simulink model "polygone_task"  (R2016a)
settings: Solver=FixedStepAuto  StartTime=0.0  StopTime=inf  FixedStep=1  RelTol=1e-3
undefined symbols (not defined in the file): Header
libraries: robotlib x3
settings Model: Creator=root  LastModifiedBy=root
settings OptimizationCC: OptimizeModelRefInitCode=on  LifeSpan=Inf  MaxStackSize=64
settings HardwareCC: ProdBitPerPointer=32  ProdLargestAtomicFloat=None  ProdIntDivRoundTo=Undefined  ProdEndianess=Unspecified  ProdWordSize=32  ProdHWDeviceType=Generic->Unspecified (assume 32-bit Generic)
settings RTWCC: SystemTargetFile=ert.tlc  HardwareBoard=Robot Operating System (ROS)  TemplateMakefile=ert_default_tmf  GenerateReport=on  Toolchain=Catkin  IncludeHyperlinkInReport=on  LaunchReport=on  TargetLang=C++  GenerateTraceInfo=on  GenerateTraceReport=on  GenerateTraceReportSl=on  GenerateTraceReportSf=on  GenerateTraceReportEml=on
settings CodeAppCC: ForceParamTrailComments=on  IgnoreCustomStorageClasses=off  OperatorAnnotations=on  SimulinkDataObjDesc=on  SFDataObjDesc=on  MATLABFcnDesc=on  InsertBlockDesc=on  MATLABSourceComments=on

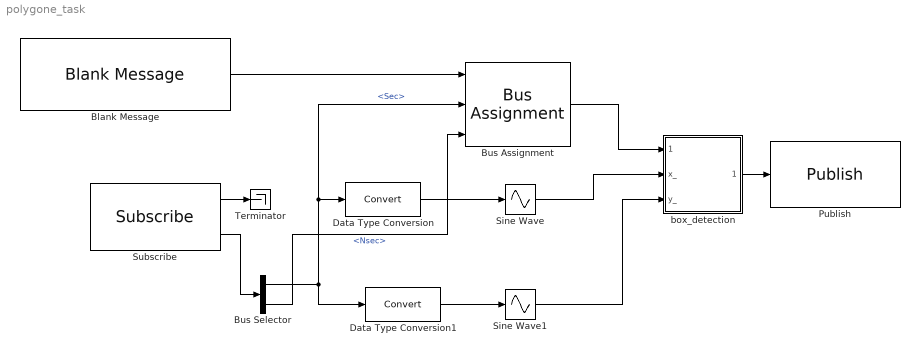
== system polygone_task ==
  Blank Message : robotlib/Blank Message  SourceLibraryInfo=This block requires Robotics System Toolbox  messageType=geometry_msgs/PolygonStamped  SampleTime=inf
  Bus Assignment : BusAssignment  AssignedSignals=Header.Stamp.Sec,Header.Stamp.Nsec
  Bus Selector : BusSelector  OutputSignals=Clock_.Sec,Clock_.Nsec
  Data Type Conversion : DataTypeConversion
  Data Type Conversion1 : DataTypeConversion
  Publish : robotlib/Publish  SourceLibraryInfo=This block requires Robotics System Toolbox  topicSource=Specify your own  topic=/detections  messageType=geometry_msgs/PolygonStamped  messageQueueLength=1
  Sine Wave : Sin  TimeSource=Use external signal  Amplitude=3  Frequency=0.2  SampleTime=0
  Sine Wave1 : Sin  TimeSource=Use external signal  Amplitude=3  Frequency=0.2  Phase=pi/2  SampleTime=0
  Subscribe : robotlib/Subscribe  SourceLibraryInfo=This block requires Robotics System Toolbox  topicSource=Specify your own  topic=/clock  messageType=rosgraph_msgs/Clock  sampleTime=-1  messageQueueLength=1
  Terminator : Terminator
  box_detection : MATLAB Function  TreatAsAtomicUnit=on
  wires:
  Subscribe/1 -> Terminator/1
  Subscribe/2 -> Bus Selector/1
  Blank Message/1 -> Bus Assignment/1
  Bus Selector/1 -> Data Type Conversion/1, Bus Assignment/2, Data Type Conversion1/1  "<Sec>"
  Bus Selector/2 -> Bus Assignment/3  "<Nsec>"
  Data Type Conversion1/1 -> Sine Wave1/1
  Data Type Conversion/1 -> Sine Wave/1
  Bus Assignment/1 -> box_detection/1(blankMsg)
  Sine Wave/1 -> box_detection/2(x_)
  Sine Wave1/1 -> box_detection/3(y_)
  box_detection/1(outputMsg) -> Publish/1

== matlab function polygone_task/box_detection ==
  data: blankMsg input; outputMsg output Bus: SL_Bus_polygone_task_geometry_msgs_PolygonStamped; x_ input; y_ input
function outputMsg = fcn(blankMsg, x_,y_)
%#codegen

persistent seq;

if isempty(seq)
    seq=uint32(0);
end

seq = seq +1;
outputMsg = blankMsg;
x = single(x_);
y = single(y_);
z = single(0);

outputMsg.Polygon.Points_SL_Info.CurrentLength = uint32(5);
str = 'catvehicle/odom';
% initialize the header and set its values
strLength = length(str);
outputMsg.Header.Seq = seq;
outputMsg.Header.FrameId(1:strLength) = str;
outputMsg.Header.FrameId_SL_Info.CurrentLength = uint32(strLength);

% populate point 1
outputMsg.Polygon.Points(1).X = floor(x);
outputMsg.Polygon.Points(1).Y = floor(y);
outputMsg.Polygon.Points(1).Z = z;

% populate point 2
outputMsg.Polygon.Points(2).X = floor(x);
outputMsg.Polygon.Points(2).Y = ceil(y);
outputMsg.Polygon.Points(2).Z = z;

% populate point 3
outputMsg.Polygon.Points(3).X = ceil(x);
outputMsg.Polygon.Points(3).Y = ceil(y);
outputMsg.Polygon.Points(3).Z = z;

% populate point 4
outputMsg.Polygon.Points(4).X = ceil(x);
outputMsg.Polygon.Points(4).Y = floor(y);
outputMsg.Polygon.Points(4).Z = z;

% populate point 5
outputMsg.Polygon.Points(4).X = ceil(x*x);
outputMsg.Polygon.Points(4).Y = floor(y/2);
outputMsg.Polygon.Points(4).Z = z;
